simulink model "Lukemia_controller"  (R2024a)
settings: Solver=VariableStepAuto  StartTime=0.0  StopTime=20  RelTol=1e-3
settings Model: Creator=samad  LastModifiedBy=samad

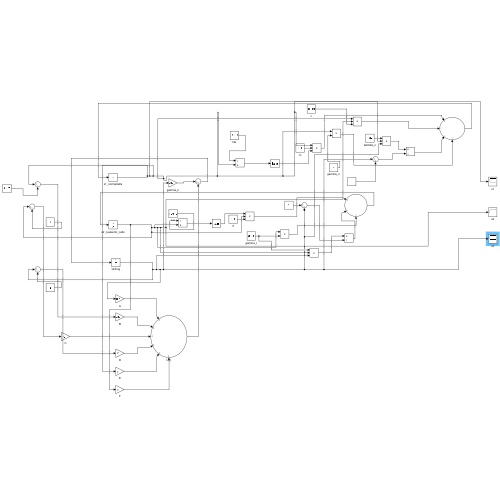
[thumbnail: Simulink's stored preview of the top-level diagram]
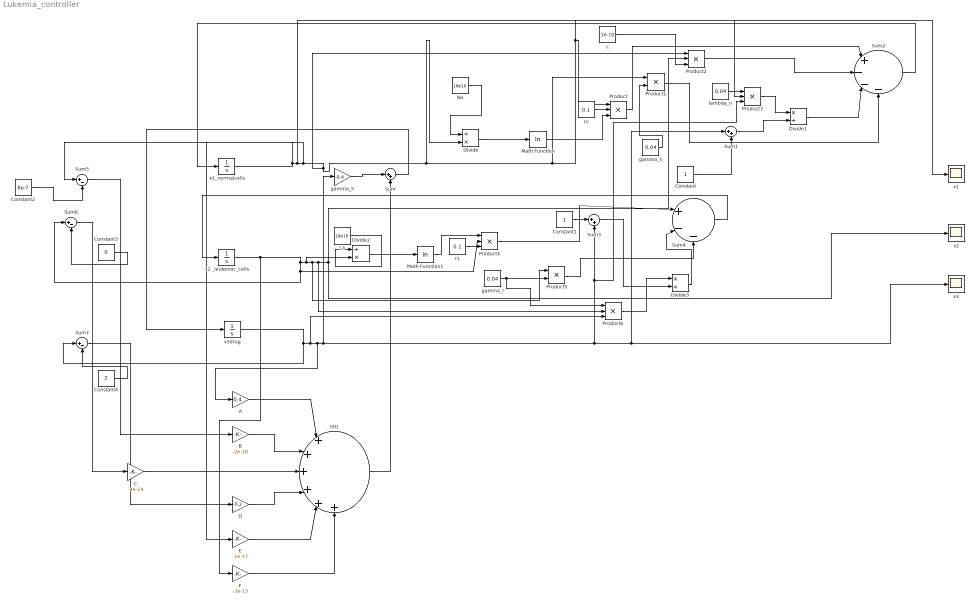
== system Lukemia_controller ==
  A : Gain  Gain=0.4
  B : Gain  Gain=-2e-18
  C : Gain  Gain=-4e-14
  Constant : Constant
  Constant1 : Constant
  Constant2 : Constant  Value=8e-7
  Constant3 : Constant  Value=0
  Constant4 : Constant  Value=2
  D : Gain  Gain=-0.2
  Divide : Product  Inputs=/*
  Divide1 : Product  Inputs=*/
  Divide2 : Product  Inputs=/*
  Divide3 : Product  Inputs=*/
  E : Gain  Gain=-1e-17
  F : Gain  Gain=-2e-13
  La : Constant  Value=10e10
  Math Function : Math  Operator=log
  Math Function1 : Math  Operator=log
  Na : Constant  Value=10e10
  Product{,2..4,6} (5 alike) : Product  Inputs=3
  Product1 : Product
  Product5 : Product
  Sum : Sum  Inputs=|++
  Sum1 : Sum  Inputs=|++
  Sum2 : Sum  Inputs=|+---
  Sum3 : Sum  Inputs=|++
  Sum4 : Sum  Inputs=|+--
  Sum5 : Sum  Inputs=|+-
  Sum6 : Sum  Inputs=|+-
  Sum7 : Sum  Inputs=|+-
  U(t) : Sum  Inputs=|++++++
  c : Constant  Value=1e-10
  gamma_h : Gain  Gain=-0.4
  gamma_l : Constant  Value=0.04
  gamma_n : Constant  Value=0.04
  lambda_n : Constant  Value=0.04
  r1 : Constant  Value=0.1
  rn : Constant  Value=0.1
  x1 : Scope
  x1_normalcells : Integrator  InitialCondition=10e8
  x2 : Scope
  x2 _leukemic_cells : Integrator  InitialCondition=1.8e8
  x3 : Scope
  x3drug : Integrator
  wires:
  U(t)/1 -> Sum/2
  Sum/1 -> x3drug/1
  Na/1 -> Divide/1
  x1_normalcells/1 -> E/1, x1/1, Sum5/1, Product3/2, Product/1, Product1/1, Divide/2, Product2/1
  Divide/1 -> Math Function/1
  rn/1 -> Product/2
  Math Function/1 -> Product/3
  gamma_n/1 -> Product1/2
  c/1 -> Product2/3
  x3drug/1 -> Sum7/1, Product6/3, A/1, x3/1, Sum1/1, Product3/3, Sum3/2, gamma_h/1
  Constant/1 -> Sum1/2
  lambda_n/1 -> Product3/1
  Product3/1 -> Divide1/1
  Sum1/1 -> Divide1/2
  Product/1 -> Sum2/1
  Product2/1 -> Sum2/2
  Divide1/1 -> Sum2/3
  Product1/1 -> Sum2/4
  Sum2/1 -> x1_normalcells/1
  La/1 -> Divide2/1
  Divide2/1 -> Math Function1/1
  Math Function1/1 -> Product4/1
  r1/1 -> Product4/3
  gamma_l/1 -> Product6/1, Product5/2
  Constant1/1 -> Sum3/1
  Product6/1 -> Divide3/1
  Sum3/1 -> Divide3/2
  gamma_h/1 -> Sum/1
  Product4/1 -> Sum4/1
  Divide3/1 -> Sum4/2
  Product5/1 -> Sum4/3
  Sum4/1 -> x2 _leukemic_cells/1
  Constant2/1 -> Sum5/2
  x2 _leukemic_cells/1 -> F/1, Sum6/1, Product4/2, Divide2/2, Product5/1, Product6/2, x2/1, Product2/2
  Constant3/1 -> Sum6/2
  Constant4/1 -> Sum7/2
  Sum5/1 -> B/1
  Sum6/1 -> C/1
  Sum7/1 -> D/1
  A/1 -> U(t)/1
  B/1 -> U(t)/2
  C/1 -> U(t)/3
  D/1 -> U(t)/4
  E/1 -> U(t)/5
  F/1 -> U(t)/6
